simulink model "Question17(a)_PD_22129011"  (R2022a)
settings: Solver=ode3  StartTime=0.0  StopTime=0.5  FixedStep=T  RelTol=1e-3
InitFcn:
  | T=5e-6
  | fsw=1550
  | Ts=1/fsw
libraries: spsIGBTDiodeLib x24, simulink x12, spsDCVoltageSourceLib x6, spsVoltageMeasurementLib x5, spsSeriesRLCBranchLib x1, spspowerguiLib x1
settings Model: Creator=ARAVINDASAI BURA  LastModifiedBy=ARAVINDASAI BURA
settings DataIOCC: SaveFormat=StructureWithTime  ReturnWorkspaceOutputs=off
settings OptimizationCC: DefaultUnderspecifiedDataType=single

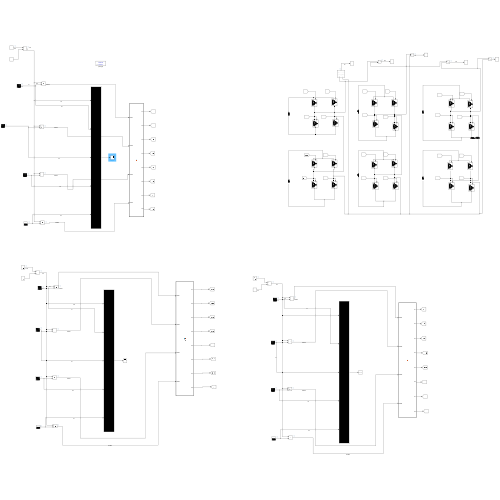
[thumbnail: Simulink's stored preview of the top-level diagram]
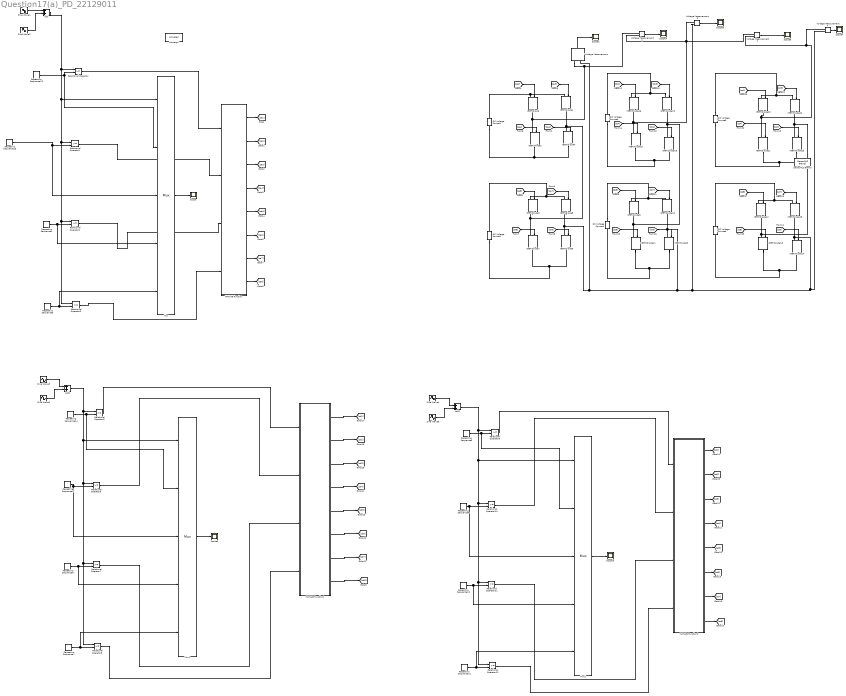
== system Question17(a)_PD_22129011 ==
  Add : Sum
  Add1 : Sum
  Add2 : Sum
  DC Voltage Source{1..6} (6 alike) : spsDCVoltageSourceLib/DC Voltage Source  Amplitude=100  Measurements=None
  IGBT/Diode{,1..23} (24 alike) : spsIGBTDiodeLib/IGBT//Diode  Ron=1e-3  Rs=1e5  Cs=inf  Measurements=off
  MATLAB Function : MATLAB Function  TreatAsAtomicUnit=on
  MATLAB Function1 : MATLAB Function  TreatAsAtomicUnit=on
  MATLAB Function2 : MATLAB Function  TreatAsAtomicUnit=on
  Mux : Mux  Inputs=5
  Mux1 : Mux  Inputs=5
  Mux2 : Mux  Inputs=5
  Relational Operator{,1..3,5..12} (12 alike) : RelationalOperator  OutDataTypeStr=boolean  RndMeth=Simplest  InputSameDT=off
  Repeating Sequence1 : simulink/Sources/Repeating Sequence  rep_seq_t=[0 1/2 1]*Ts  rep_seq_y=[0 0.5 0]
  Repeating Sequence10 : simulink/Sources/Repeating Sequence  rep_seq_t=[0 1/2 1]*Ts  rep_seq_y=[-0.5 0 -0.5]
  Repeating Sequence11 : simulink/Sources/Repeating Sequence  rep_seq_t=[0 1/2 1]*Ts  rep_seq_y=[-1 -0.5 -1]
  Repeating Sequence12 : simulink/Sources/Repeating Sequence  rep_seq_t=[0 1/2 1]*Ts  rep_seq_y=[0.5 1 0.5]
  Repeating Sequence13 : simulink/Sources/Repeating Sequence  rep_seq_t=[0 1/2 1]*Ts  rep_seq_y=[0 0.5 0]
  Repeating Sequence14 : simulink/Sources/Repeating Sequence  rep_seq_t=[0 1/2 1]*Ts  rep_seq_y=[0.5 1 0.5]
  Repeating Sequence2 : simulink/Sources/Repeating Sequence  rep_seq_t=[0 1/2 1]*Ts  rep_seq_y=[-0.5 0 -0.5]
  Repeating Sequence3 : simulink/Sources/Repeating Sequence  rep_seq_t=[0 1/2 1]*Ts  rep_seq_y=[-1 -0.5 -1]
  Repeating Sequence4 : simulink/Sources/Repeating Sequence  rep_seq_t=[0 1/2 1]*Ts  rep_seq_y=[0 0.5 0]
  Repeating Sequence5 : simulink/Sources/Repeating Sequence  rep_seq_t=[0 1/2 1]*Ts  rep_seq_y=[0.5 1 0.5]
  Repeating Sequence6 : simulink/Sources/Repeating Sequence  rep_seq_t=[0 1/2 1]*Ts  rep_seq_y=[-0.5 0 -0.5]
  Repeating Sequence7 : simulink/Sources/Repeating Sequence  rep_seq_t=[0 1/2 1]*Ts  rep_seq_y=[-1 -0.5 -1]
  Scope{,1..7} (8 alike) : Scope
  Series RLC Branch : spsSeriesRLCBranchLib/Series RLC Branch  LConnTagsString=__new0  RConnTagsString=__new0  BranchType=RL  Resistance=10  Inductance=50e-3  SetiL0=off  InitialCurrent=0  Capacitance=1e-6  Setx0=off  InitialVoltage=0  Measurements=None
  Sine Wave1 : Sin  Amplitude=1.15  Frequency=2*pi*50  SampleTime=0
  Sine Wave2 : Sin  Amplitude=1.15/6  Frequency=2*pi*50*3  SampleTime=0
  Sine Wave3 : Sin  Amplitude=1.15  Frequency=2*pi*50  Phase=-(2/3)*pi  SampleTime=0
  Sine Wave4 : Sin  Amplitude=1.15  Frequency=2*pi*50  Phase=-(4/3)*pi  SampleTime=0
  Sine Wave5 : Sin  Amplitude=1.15/6  Frequency=2*pi*50*3  SampleTime=0
  Sine Wave6 : Sin  Amplitude=1.15/6  Frequency=2*pi*50*3  SampleTime=0
  Voltage Measurement{,1..4} (5 alike) : spsVoltageMeasurementLib/Voltage Measurement  PhasorSimulation=off  OutputType=Complex  PSBequivalent=0
  powergui : spspowerguiLib/powergui  Priority=1  SimulationMode=Discrete  SampleTime=5e-6  frequency=60  Iterations=50  frequencyindice=0  Pbase=100e6  ErrMax=1e-4  UnitsV=kV  UnitsW=MW  buscounter=0  FunctionMessages=off  echomessages=off  EnableUseOfTLC=off  CurrentSourceSwitches=off  DisableSnubberDevices=off  DisableRonSwitches=off  DisableVfSwitches=off  DisplayEquations=off  AutomaticDiscreteSolvers=off  SolverType=Tustin/Backward Euler (TBE)  Interpol=off  ExternalGateDelay=off  methode=off  Ts=100  x0status=blocks  SPID=on  SwTol=0  HookPort=off  NonlinearTolerance=1e-4  nMaxIteration=100  ContinueOnMaxIteration=off  RestoreLinks=warning  ResistiveCurrentMeasurement=off  Frange=[0:2:500]  Ylog=off  Xlog=on  ShowGrid=off  save=off  variable=ZData  structure=0  ZoomFFT=off  StartTime=0.0  cycles=1  DisplayStyle=1  fundamental=60  FreqAxis=off  MaxFrequency=1000  frequencyindicesteady=1  RmsSteady=1  display=off
  wires:
  [sa5] -> IGBT/Diode3/1
  [sa4] -> IGBT/Diode2/1
  [sa7] -> IGBT/Diode5/1
  [sa2] -> IGBT/Diode4/1
  [sa1] -> IGBT/Diode/1
  [sa3] -> IGBT/Diode1/1
  [sa6] -> IGBT/Diode6/1
  [sa8] -> IGBT/Diode7/1
  [sb7] -> IGBT/Diode10/1
  [sb6] -> IGBT/Diode9/1
  [sb2] -> IGBT/Diode18/1
  [sb4] -> IGBT/Diode17/1
  [sb5] -> IGBT/Diode8/1
  [sb3] -> IGBT/Diode19/1
  [sb1] -> IGBT/Diode16/1
  [sb8] -> IGBT/Diode11/1
  [sc6] -> IGBT/Diode14/1
  [sc2] -> IGBT/Diode23/1
  [sc4] -> IGBT/Diode21/1
  [sc5] -> IGBT/Diode12/1
  [sc3] -> IGBT/Diode22/1
  [sc1] -> IGBT/Diode20/1
  [sc8] -> IGBT/Diode13/1
  Repeating Sequence13/1 -> Mux/3, Relational Operator1/2  "ca2"
  Repeating Sequence2/1 -> Mux/4, Relational Operator2/2  "ca3"
  Add/1 -> Mux/1, Relational Operator3/1, Relational Operator2/1, Relational Operator1/1, Relational Operator/1  "sina"
  Repeating Sequence3/1 -> Mux/5, Relational Operator3/2  "ca4"
  Relational Operator/1 -> MATLAB Function/1(PWM1)  "PWMa1"
  Relational Operator2/1 -> MATLAB Function/3(PWM3)  "PWMa3"
  Relational Operator3/1 -> MATLAB Function/4(PWM4)  "PWMa4"
  Mux/1 -> Scope/1
  Relational Operator1/1 -> MATLAB Function/2(PWM2)  "PWMa2"
  MATLAB Function/1(sa1) -> [sa1]
  MATLAB Function/2(sa2) -> [sa2]
  MATLAB Function/3(sa3) -> [sa3]
  MATLAB Function/4(sa4) -> [sa4]
  MATLAB Function/6(sa6) -> [sa6]
  MATLAB Function/7(sa7) -> [sa7]
  MATLAB Function/8(sa8) -> [sa8]
  MATLAB Function2/8(sc8) -> [sc8]
  MATLAB Function1/8(sb8) -> [sb8]
  MATLAB Function1/7(sb7) -> [sb7]
  MATLAB Function1/6(sb6) -> [sb6]
  MATLAB Function1/5(sb5) -> [sb5]
  MATLAB Function1/4(sb4) -> [sb4]
  MATLAB Function1/3(sb3) -> [sb3]
  MATLAB Function1/2(sb2) -> [sb2]
  MATLAB Function1/1(sb1) -> [sb1]
  MATLAB Function2/1(sc1) -> [sc1]
  MATLAB Function2/2(sc2) -> [sc2]
  MATLAB Function2/3(sc3) -> [sc3]
  MATLAB Function2/4(sc4) -> [sc4]
  MATLAB Function2/5(sc5) -> [sc5]
  MATLAB Function2/6(sc6) -> [sc6]
  MATLAB Function2/7(sc7) -> [sc7]
  Voltage Measurement/1 -> Scope1/1  "Van"
  Mux1/1 -> Scope2/1
  Relational Operator7/1 -> MATLAB Function1/3(PWM3)  "PWMb3"
  Relational Operator8/1 -> MATLAB Function1/4(PWM4)  "PWMb4"
  Repeating Sequence1/1 -> Mux1/3, Relational Operator6/2  "cb2"
  Repeating Sequence14/1 -> Mux1/2, Relational Operator5/2  "cb1"
  Repeating Sequence7/1 -> Mux1/5, Relational Operator8/2  "cb4"
  Relational Operator5/1 -> MATLAB Function1/1(PWM1)  "PWMb1"
  Add1/1 -> Relational Operator8/1, Relational Operator7/1, Relational Operator6/1, Mux1/1, Relational Operator5/1  "sinb"
  Repeating Sequence6/1 -> Mux1/4, Relational Operator7/2  "cb3"
  Relational Operator6/1 -> MATLAB Function1/2(PWM2)  "PWMb2"
  Mux2/1 -> Scope3/1
  Relational Operator11/1 -> MATLAB Function2/3(PWM3)  "PWMc3"
  Relational Operator12/1 -> MATLAB Function2/4(PWM4)  "PWMc4"
  Repeating Sequence4/1 -> Mux2/3, Relational Operator10/2  "cc2"
  Repeating Sequence5/1 -> Mux2/2, Relational Operator9/2  "cc1"
  Repeating Sequence11/1 -> Mux2/5, Relational Operator12/2  "cc4"
  Relational Operator9/1 -> MATLAB Function2/1(PWM1)  "PWMc1"
  Add2/1 -> Relational Operator12/1, Relational Operator11/1, Relational Operator10/1, Mux2/1, Relational Operator9/1  "sinc"
  Repeating Sequence10/1 -> Mux2/4, Relational Operator11/2  "cc3"
  Relational Operator10/1 -> MATLAB Function2/2(PWM2)  "PWMc2"
  MATLAB Function/5(sa5) -> [sa5]
  Sine Wave2/1 -> Add/2  "sine"
  Sine Wave5/1 -> Add1/2  "sine"
  Sine Wave3/1 -> Add1/1  "sinbb"
  Sine Wave6/1 -> Add2/2  "sine"
  Sine Wave4/1 -> Add2/1  "sincc"
  [sc7] -> IGBT/Diode15/1
  Voltage Measurement1/1 -> Scope4/1  "Vab"
  Voltage Measurement2/1 -> Scope5/1  "Vbc"
  Repeating Sequence12/1 -> Relational Operator/2, Mux/2  "ca1"
  Voltage Measurement3/1 -> Scope6/1  "Vbn"
  Voltage Measurement4/1 -> Scope7/1  "Vcn"
  Sine Wave1/1 -> Add/1  "sina"
  connections:
  DC Voltage Source5/RConn1 -- IGBT/Diode22/LConn1 -- IGBT/Diode20/LConn1
  Voltage Measurement/LConn1 -- Voltage Measurement1/LConn1 -- IGBT/Diode2/LConn1 -- IGBT/Diode/RConn1
  DC Voltage Source4/RConn1 -- IGBT/Diode10/LConn1 -- IGBT/Diode8/LConn1
  IGBT/Diode4/LConn1 -- IGBT/Diode1/RConn1 -- IGBT/Diode7/LConn1 -- IGBT/Diode3/RConn1
  DC Voltage Source4/LConn1 -- IGBT/Diode11/RConn1 -- IGBT/Diode9/RConn1
  IGBT/Diode16/RConn1 -- Voltage Measurement3/LConn1 -- Voltage Measurement1/LConn2 -- Voltage Measurement2/LConn1 -- IGBT/Diode17/LConn1
  IGBT/Diode19/RConn1 -- IGBT/Diode18/LConn1 -- IGBT/Diode11/LConn1 -- IGBT/Diode8/RConn1
  IGBT/Diode20/RConn1 -- IGBT/Diode21/LConn1 -- Voltage Measurement4/LConn1 -- Voltage Measurement2/LConn2
  IGBT/Diode23/LConn1 -- IGBT/Diode22/RConn1 -- IGBT/Diode12/RConn1 -- IGBT/Diode13/LConn1
  IGBT/Diode23/RConn1 -- DC Voltage Source5/LConn1 -- IGBT/Diode21/RConn1
  IGBT/Diode5/RConn1 -- IGBT/Diode6/LConn1 -- IGBT/Diode9/LConn1 -- IGBT/Diode10/RConn1 -- Voltage Measurement3/LConn2 -- Voltage Measurement4/LConn2 -- IGBT/Diode15/RConn1 -- IGBT/Diode14/LConn1 -- Voltage Measurement/LConn2
  IGBT/Diode19/LConn1 -- DC Voltage Source3/RConn1 -- IGBT/Diode16/LConn1
  IGBT/Diode17/RConn1 -- DC Voltage Source3/LConn1 -- IGBT/Diode18/RConn1
  DC Voltage Source1/LConn1 -- IGBT/Diode4/RConn1 -- IGBT/Diode2/RConn1
  DC Voltage Source1/RConn1 -- IGBT/Diode1/LConn1 -- IGBT/Diode/LConn1
  IGBT/Diode7/RConn1 -- DC Voltage Source2/LConn1 -- IGBT/Diode6/RConn1
  IGBT/Diode5/LConn1 -- DC Voltage Source2/RConn1 -- IGBT/Diode3/LConn1
  IGBT/Diode13/RConn1 -- DC Voltage Source6/LConn1 -- IGBT/Diode14/RConn1
  DC Voltage Source6/RConn1 -- IGBT/Diode15/LConn1 -- IGBT/Diode12/LConn1

== matlab function Question17(a)_PD_22129011/MATLAB Function1 ==
  data: PWM1 input; sb1 output; PWM2 input; PWM3 input; PWM4 input; sb2 output; sb3 output; sb4 output; sb5 output; sb6 output; sb7 output; sb8 output
function [sb1,sb2,sb3,sb4,sb5,sb6,sb7,sb8] = fcn(PWM1,PWM2,PWM3,PWM4)
sum=PWM1+PWM2+PWM3+PWM4;
sb1=0;
sb2=0;
sb3=0;
sb4=0;
sb5=0;
sb6=0;
sb7=0;
sb8=0;
if(sum==4) %Va0=2Vdc
    sb1=1;
    sb2=1;
    sb3=0;
    sb4=0;
    sb5=1;
    sb6=1;
    sb7=0;
    sb8=0;
elseif(sum==3)%Vao=Vdc
    sb1=1;
    sb2=1;
    sb3=0;
    sb4=0;
    sb5=1;
    sb6=0;
    sb7=1;
    sb8=0;
elseif(sum==2)%Vao=0
    sb1=1;
    sb2=0;
    sb3=1;
    sb4=0;
    sb5=1;
    sb6=0;
    sb7=1;
    sb8=0;
elseif(sum==1)%Vao=-Vdc
    sb1=0;
    sb2=0;
    sb3=1;
    sb4=1;
    sb5=1;
    sb6=0;
    sb7=1;
    sb8=0;
elseif(sum==0)%Vao=-2Vdc
    sb1=0;
    sb2=0;
    sb3=1;
    sb4=1;
    sb5=0;
    sb6=0;
    sb7=1;
    sb8=1;
end
end

== matlab function Question17(a)_PD_22129011/MATLAB Function ==
  data: PWM1 input; sa1 output; PWM2 input; PWM3 input; PWM4 input; sa2 output; sa3 output; sa4 output; sa5 output; sa6 output; sa7 output; sa8 output
function [sa1,sa2,sa3,sa4,sa5,sa6,sa7,sa8] = fcn(PWM1,PWM2,PWM3,PWM4)
sum=PWM1+PWM2+PWM3+PWM4;
sa1=0;
sa2=0;
sa3=0;
sa4=0;
sa5=0;
sa6=0;
sa7=0;
sa8=0;
if(sum==4) %Va0=2Vdc
    sa1=1;
    sa2=1;
    sa3=0;
    sa4=0;
    sa5=1;
    sa6=1;
    sa7=0;
    sa8=0;
elseif(sum==3)%Vao=Vdc
    sa1=1;
    sa2=1;
    sa3=0;
    sa4=0;
    sa5=1;
    sa6=0;
    sa7=1;
    sa8=0;
elseif(sum==2)%Vao=0
    sa1=1;
    sa2=0;
    sa3=1;
    sa4=0;
    sa5=1;
    sa6=0;
    sa7=1;
    sa8=0;
elseif(sum==1)%Vao=-Vdc
    sa1=0;
    sa2=0;
    sa3=1;
    sa4=1;
    sa5=1;
    sa6=0;
    sa7=1;
    sa8=0;
elseif(sum==0)%Vao=-2Vdc
    sa1=0;
    sa2=0;
    sa3=1;
    sa4=1;
    sa5=0;
    sa6=0;
    sa7=1;
    sa8=1;
end
end

== matlab function Question17(a)_PD_22129011/MATLAB Function2 ==
  data: PWM1 input; sc1 output; PWM2 input; PWM3 input; PWM4 input; sc2 output; sc3 output; sc4 output; sc5 output; sc6 output; sc7 output; sc8 output
function [sc1,sc2,sc3,sc4,sc5,sc6,sc7,sc8] = fcn(PWM1,PWM2,PWM3,PWM4)
sum=PWM1+PWM2+PWM3+PWM4;
sc1=0;
sc2=0;
sc3=0;
sc4=0;
sc5=0;
sc6=0;
sc7=0;
sc8=0;
if(sum==4) %Va0=2Vdc
    sc1=1;
    sc2=1;
    sc3=0;
    sc4=0;
    sc5=1;
    sc6=1;
    sc7=0;
    sc8=0;
elseif(sum==3)%Vao=Vdc
    sc1=1;
    sc2=1;
    sc3=0;
    sc4=0;
    sc5=1;
    sc6=0;
    sc7=1;
    sc8=0;
elseif(sum==2)%Vao=0
    sc1=1;
    sc2=0;
    sc3=1;
    sc4=0;
    sc5=1;
    sc6=0;
    sc7=1;
    sc8=0;
elseif(sum==1)%Vao=-Vdc
    sc1=0;
    sc2=0;
    sc3=1;
    sc4=1;
    sc5=1;
    sc6=0;
    sc7=1;
    sc8=0;
elseif(sum==0)%Vao=-2Vdc
    sc1=0;
    sc2=0;
    sc3=1;
    sc4=1;
    sc5=0;
    sc6=0;
    sc7=1;
    sc8=1;
end
end
